simulink model "Lab1T2"  (R2018b)
settings: Solver=VariableStepAuto  StartTime=0.0  StopTime=100  RelTol=1e-3
settings Model: Creator=aloisia  LastModifiedBy=aloisia
settings SFSimCC: SimUseLocalCustomCode=off
settings RTWCC: RTWUseLocalCustomCode=off

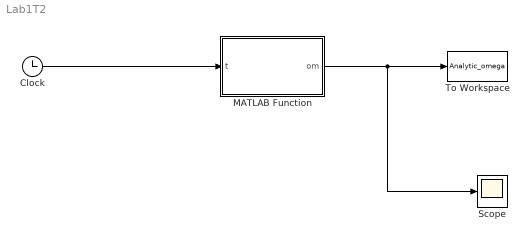
== system Lab1T2 ==
  Clock : Clock
      settings: Decimation=500
  MATLAB Function : MATLAB Function  TreatAsAtomicUnit=on
  Scope : Scope
  To Workspace : ToWorkspace  VariableName=Analytic_omega  SaveFormat=Timeseries  SampleTime=-1
  wires:
  Clock/1 -> MATLAB Function/1(t)
  MATLAB Function/1(om) -> Scope/1, To Workspace/1

== matlab function Lab1T2/MATLAB Function ==
  data: om output; t input
function om = Analytic_Euler(t)

om_0 = [0.45; 0.55; 0.52];
Ix = 0.07; %[kgm^2]
Iy = 0.0504; %[kgm^2]
Iz = 0.0109; %[kgm^2]

lambda = (Iz -Ix)/Ix * om_0(3);
om = zeros(3,1);

om(1) = om_0(1)*cos(lambda*t) - om_0(2)*sin(lambda*t);
om(2) = om_0(1)*sin(lambda*t) + om_0(2)*cos(lambda*t);
om(3) = om_0(3);

end
